simulink model "Lab8(1)"  (R2022a)
settings: Solver=ode45  StartTime=0.0  StopTime=3  RelTol=1e-3
values from neighbouring files (symbols this model uses):
  Beq = Bm +Bl/N^2    (= 0)    [VarBode_2.m]    (also in VarLab8(1).m)
  degs2rpm = 60/360    (= 0.166666666667)    [VarLab8(1).m]
  Jeq = Jm + Jl/N^2    (= 5.50204081633e-07)    [VarBode_2.m]    (also in VarLab8(1).m)
  Ki = 17.71    [VarLab8(1).m]
  KpP = 1    [VarLab8(1).m]
  KpPI = 0.22    [VarLab8(1).m]
  Kw = 1/Tw    (= 33.3333333333)    [VarLab8(1).m]
  N = 14    [VarBode_2.m]    (also in VarLab8(1).m)
  rads2rpm = 60/2/pi    (= 9.54929658551)    [VarLab8(1).m]
  Req = Ra + Rs    (= 3.1)    [VarBode_2.m]    (also in VarLab8(1).m)
  rpm2rads = 2*pi/60    (= 0.10471975512)    [VarLab8(1).m]
  Tausf = 0.0098    [VarLab8(1).m]
  Tc = 1/(2*pi*50)    (= 0.00318309886184)    [VarLab8(1).m]
  Ts = 4e-3    (= 0.004)    [VarLab8(1).m]
undefined symbols (not defined in the file or in its folder): daq, denH, DiscIntNeverNeededParam, drv, gbox, mld, mot, numH, sens
settings Model: Creator=bonvoltnuovo  LastModifiedBy=bonaventur
settings SolverCC: ZeroCrossAlgorithm=Adaptive
settings DebuggingCC: IgnoredZcDiagnostic=none  UnconnectedInputMsg=warning  UnconnectedOutputMsg=warning  UnconnectedLineMsg=warning
settings RTWCC: DLArmComputeVersion=19.05

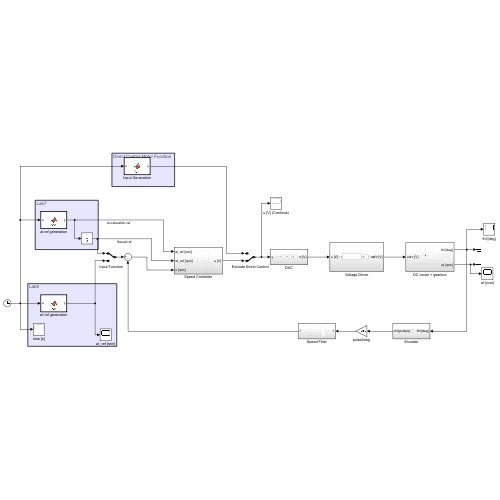
[thumbnail: Simulink's stored preview of the top-level diagram]
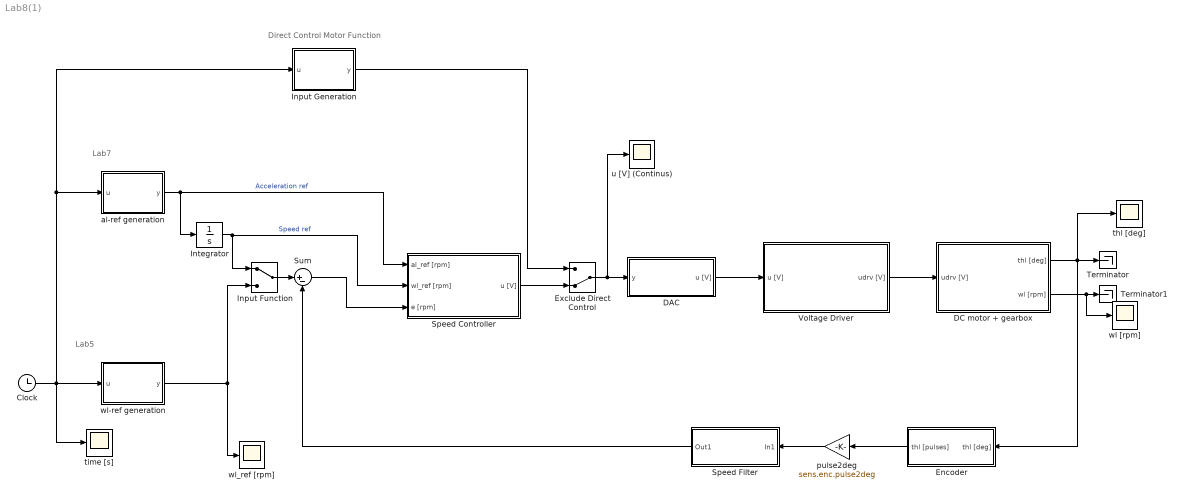
== system Lab8(1) ==
  note: Lab5
  note: Direct Control Motor Function
  note: Lab7
  Clock : Clock
  DAC : Subsystem
  DC motor + gearbox : Subsystem
  Encoder : Subsystem
  Exclude Direct Control : ManualSwitch  CurrentSetting=0
  Input Function : ManualSwitch
  Input Generation : MATLAB Function  TreatAsAtomicUnit=on
  Integrator : Integrator
  Speed Controller : Subsystem
  Speed Filter : Subsystem
  Sum : Sum  Inputs=|+-
  Terminator : Terminator
  Terminator1 : Terminator
  Voltage Driver : Subsystem
  al-ref generation : MATLAB Function  TreatAsAtomicUnit=on
  pulse2deg : Gain  Gain=sens.enc.pulse2deg
  thl [deg] : Scope
  time [s] : Scope
  u [V] (Continus) : Scope
  wl [rpm] : Scope
  wl-ref generation : MATLAB Function  TreatAsAtomicUnit=on
  wl_ref [rpm] : Scope
  wires:
  DAC/1(u [V]) -> Voltage Driver/1(u [V])
  Voltage Driver/1(udrv [V]) -> DC motor + gearbox/1(udrv [V])
  DC motor + gearbox/2(wl [rpm]) -> wl [rpm]/1, Terminator1/1
  DC motor + gearbox/1(thl [deg]) -> thl [deg]/1, Terminator/1, Encoder/1(thl [deg])
  pulse2deg/1 -> Speed Filter/1(In1)
  Encoder/1(thl [pulses]) -> pulse2deg/1
  Speed Filter/1(Out1) -> Sum/2
  Sum/1 -> Speed Controller/3(e [rpm])
  Clock/1 -> al-ref generation/1(u), Input Generation/1(u), wl-ref generation/1(u), time [s]/1
  Input Generation/1(y) -> Exclude Direct Control/1
  Exclude Direct Control/1 -> u [V] (Continus)/1, DAC/1(y)
  Speed Controller/1(u [V]) -> Exclude Direct Control/2
  wl-ref generation/1(y) -> Input Function/2, wl_ref [rpm]/1
  Input Function/1 -> Sum/1
  Integrator/1 -> Speed Controller/2(wl_ref [rpm]), Input Function/1  "Speed ref"
  al-ref generation/1(y) -> Speed Controller/1(al_ref [rpm]), Integrator/1  "Acceleration ref"

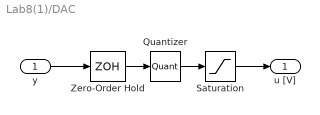
== system Lab8(1)/DAC ==
  y : Inport
  Quantizer : Quantizer  QuantizationInterval=daq.dac.q
  Saturation : Saturate  UpperLimit=daq.dac.fs  LowerLimit=-1*daq.dac.fs
  Zero-Order Hold : ZeroOrderHold  SampleTime=Ts
  u [V] : Outport
  wires:
  y/1 -> Zero-Order Hold/1
  Zero-Order Hold/1 -> Quantizer/1
  Quantizer/1 -> Saturation/1
  Saturation/1 -> u [V]/1

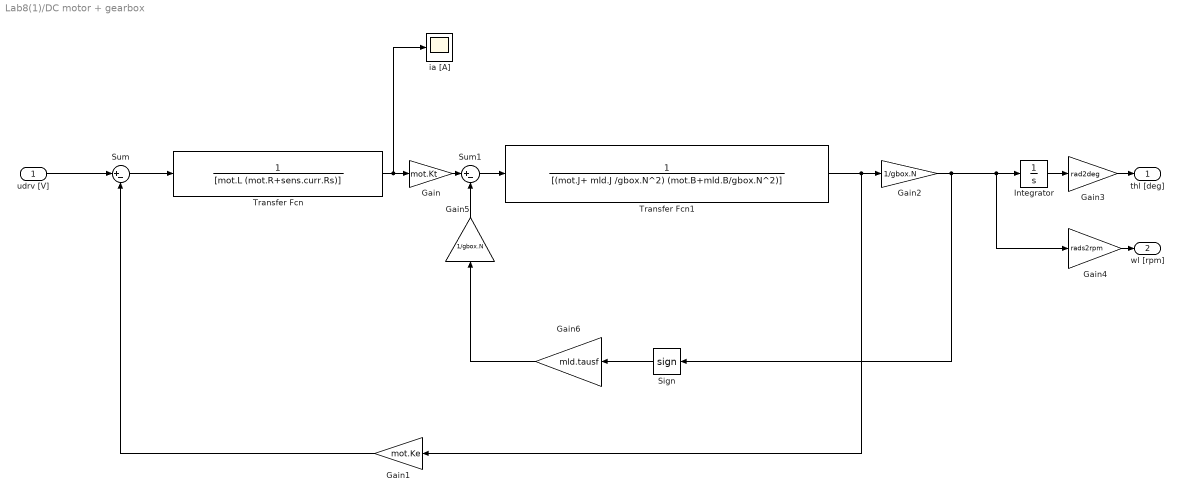
== system Lab8(1)/DC motor + gearbox ==
  udrv [V] : Inport
  Gain : Gain  Gain=mot.Kt
  Gain1 : Gain  Gain=mot.Ke
  Gain2 : Gain  Gain=1/gbox.N
  Gain3 : Gain  Gain=rad2deg
  Gain4 : Gain  Gain=rads2rpm
  Gain5 : Gain  Gain=1/gbox.N
  Gain6 : Gain  Gain=mld.tausf
  Integrator : Integrator
  Sign : Signum  ZeroCross=off
  Sum : Sum  Inputs=|+-
  Sum1 : Sum  Inputs=|+-
  Transfer Fcn : TransferFcn  Denominator=[mot.L (mot.R+sens.curr.Rs)]
  Transfer Fcn1 : TransferFcn  Denominator=[(mot.J+ mld.J /gbox.N^2) (mot.B+mld.B/gbox.N^2)]
  ia [A] : Scope
  thl [deg] : Outport
  wl [rpm] : Outport  Port=2
  wires:
  udrv [V]/1 -> Sum/1
  Gain/1 -> Sum1/1
  Transfer Fcn/1 -> ia [A]/1, Gain/1
  Sum/1 -> Transfer Fcn/1
  Sum1/1 -> Transfer Fcn1/1
  Transfer Fcn1/1 -> Gain1/1, Gain2/1
  Gain2/1 -> Gain4/1, Integrator/1, Sign/1
  Integrator/1 -> Gain3/1
  Gain3/1 -> thl [deg]/1
  Gain4/1 -> wl [rpm]/1
  Gain1/1 -> Sum/2
  Gain5/1 -> Sum1/2
  Sign/1 -> Gain6/1
  Gain6/1 -> Gain5/1

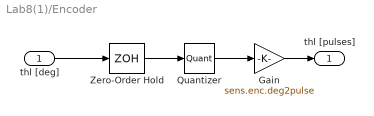
== system Lab8(1)/Encoder ==
  thl [deg] : Inport
  Gain : Gain  Gain=sens.enc.deg2pulse
  Quantizer : Quantizer  QuantizationInterval=sens.enc.pulse2deg
  Zero-Order Hold : ZeroOrderHold  SampleTime=Ts
  thl [pulses] : Outport
  wires:
  Zero-Order Hold/1 -> Quantizer/1
  Gain/1 -> thl [pulses]/1
  thl [deg]/1 -> Zero-Order Hold/1
  Quantizer/1 -> Gain/1

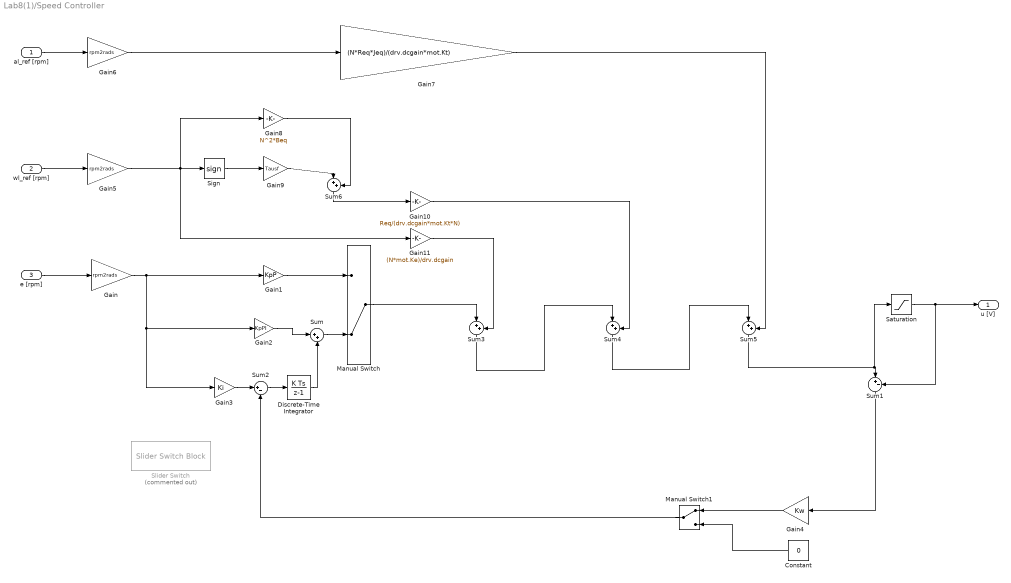
== system Lab8(1)/Speed Controller ==
  al_ref [rpm] : Inport
  wl_ref [rpm] : Inport  Port=2
  e [rpm] : Inport  Port=3
  Constant : Constant  Value=0
  Discrete-Time Integrator : DiscreteIntegrator  SampleTime=-1  ICPrevOutput=DiscIntNeverNeededParam  ICPrevScaledInput=DiscIntNeverNeededParam
  Gain : Gain  Gain=rpm2rads
  Gain1 : Gain  Gain=KpP
  Gain10 : Gain  Gain=Req/(drv.dcgain*mot.Kt*N)
  Gain11 : Gain  Gain=(N*mot.Ke)/drv.dcgain
  Gain2 : Gain  Gain=KpPI
  Gain3 : Gain  Gain=Ki
  Gain4 : Gain  Gain=Kw
  Gain5 : Gain  Gain=rpm2rads
  Gain6 : Gain  Gain=rpm2rads
  Gain7 : Gain  Gain=(N*Req*Jeq)/(drv.dcgain*mot.Kt)
  Gain8 : Gain  Gain=N^2*Beq
  Gain9 : Gain  Gain=Tausf
  Manual Switch : ManualSwitch  CurrentSetting=0
  Manual Switch1 : ManualSwitch
  Saturation : Saturate  UpperLimit=10  LowerLimit=-10
  Sign : Signum
  Slider Switch : SliderSwitchBlock  Commented=on
      settings: Values={{'Off', 'On'}, [0 1]}
  Sum{,3..6} (5 alike) : Sum  Inputs=|++
  Sum1 : Sum  Inputs=|+-
  Sum2 : Sum  Inputs=|+-
  u [V] : Outport
  wires:
  Gain/1 -> Gain3/1, Gain2/1, Gain1/1
  e [rpm]/1 -> Gain/1
  Gain1/1 -> Manual Switch/1
  Saturation/1 -> u [V]/1, Sum1/2
  Discrete-Time Integrator/1 -> Sum/2
  Sum/1 -> Manual Switch/2
  Gain2/1 -> Sum/1
  Sum1/1 -> Gain4/1
  Gain3/1 -> Sum2/1
  Sum2/1 -> Discrete-Time Integrator/1
  Gain4/1 -> Manual Switch1/1
  Manual Switch1/1 -> Sum2/2
  Constant/1 -> Manual Switch1/2
  Manual Switch/1 -> Sum3/1
  Sum3/1 -> Sum4/1
  Sum4/1 -> Sum5/1
  Sum5/1 -> Saturation/1, Sum1/1
  al_ref [rpm]/1 -> Gain6/1
  wl_ref [rpm]/1 -> Gain5/1
  Gain5/1 -> Gain11/1, Gain8/1, Sign/1
  Sign/1 -> Gain9/1
  Gain9/1 -> Sum6/1
  Gain8/1 -> Sum6/2
  Gain6/1 -> Gain7/1
  Gain11/1 -> Sum3/2
  Sum6/1 -> Gain10/1
  Gain10/1 -> Sum4/2
  Gain7/1 -> Sum5/2

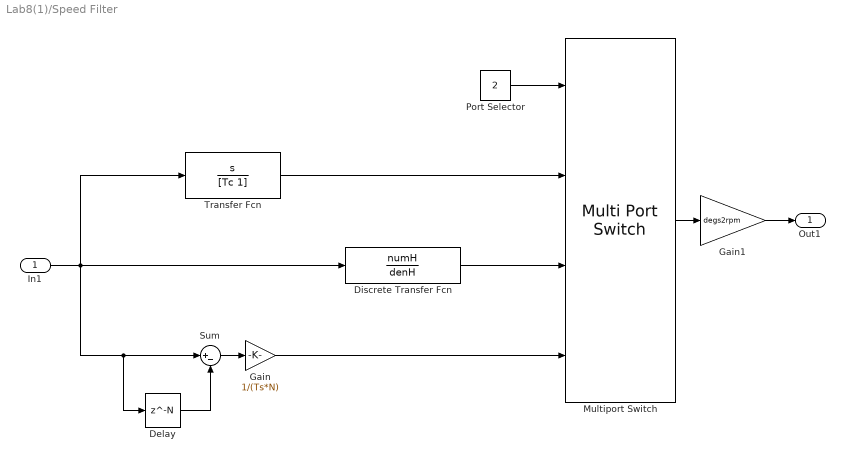
== system Lab8(1)/Speed Filter ==
  In1 : Inport
  Delay : Delay  DelayLength=N
  Discrete Transfer Fcn : DiscreteTransferFcn  Numerator=numH  Denominator=denH
  Gain : Gain  Gain=1/(Ts*N)
  Gain1 : Gain  Gain=degs2rpm
  Multiport Switch : MultiPortSwitch  SaturateOnIntegerOverflow=off  InputSameDT=off
  Port Selector : Constant  Value=2
  Sum : Sum  Inputs=|+-
  Transfer Fcn : TransferFcn  Numerator=[1 0]  Denominator=[Tc 1]
  Out1 : Outport
  wires:
  Transfer Fcn/1 -> Multiport Switch/2
  Port Selector/1 -> Multiport Switch/1
  Multiport Switch/1 -> Gain1/1
  Gain1/1 -> Out1/1
  In1/1 -> Discrete Transfer Fcn/1, Delay/1, Sum/1, Transfer Fcn/1
  Discrete Transfer Fcn/1 -> Multiport Switch/3
  Sum/1 -> Gain/1
  Delay/1 -> Sum/2
  Gain/1 -> Multiport Switch/4

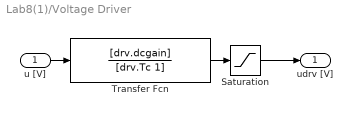
== system Lab8(1)/Voltage Driver ==
  u [V] : Inport
  Saturation : Saturate  UpperLimit=drv.outmax  LowerLimit=-1*drv.outmax
  Transfer Fcn : TransferFcn  Numerator=[drv.dcgain]  Denominator=[drv.Tc 1]
  udrv [V] : Outport
  wires:
  Saturation/1 -> udrv [V]/1
  u [V]/1 -> Transfer Fcn/1
  Transfer Fcn/1 -> Saturation/1

== matlab function Lab8(1)/wl-ref generation ==
  data: u input; y output
function y = fcn(u)
    y=0;
    if(u>=0 && u<1.5)
        y=450;
    end
    if(u>=1.5 && u<3)
        y=-450;
    end
end

== matlab function Lab8(1)/al-ref generation ==
  data: u input; y output
function y = fcn(u)
    y=0;
    if(u>=0 && u<0.5)
        y=900;
    end
    if(u>=0.5 && u<1.0)
        y=0;
    end
    if(u>=1.0 && u<2.0)
        y=-900;
    end
    if(u>=2.0 && u<2.5)
        y=0;
    end
    if(u>=2.5 && u<3.0)
        y=900;
    end 
end

== matlab function Lab8(1)/Input Generation ==
  data: u input; y output
function y = fcn(u)
    y=0;
    if(u>=0 && u<1.5)
        y=6;
    end
    if(u>=1.5 && u<3)
        y=-6;
    end
end
